simulink subsystem "dual_spin_omega_dot"  (R2023b)
settings: Solver=VariableStepAuto  StartTime=0.0  StopTime=10.0  RelTol=1e-3
libraries: matrix_library x1
settings Model: Creator=pierb  LastModifiedBy=pierb

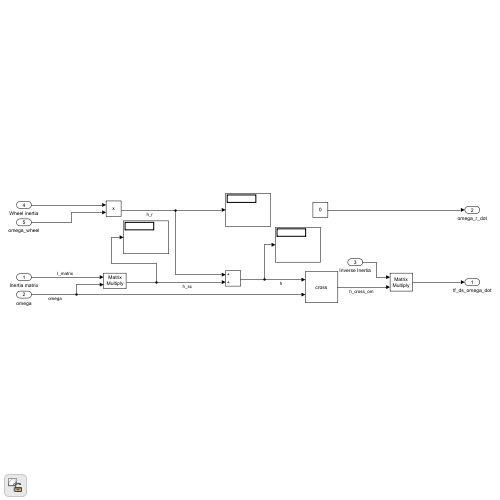
[thumbnail: Simulink's stored preview of the top-level diagram]
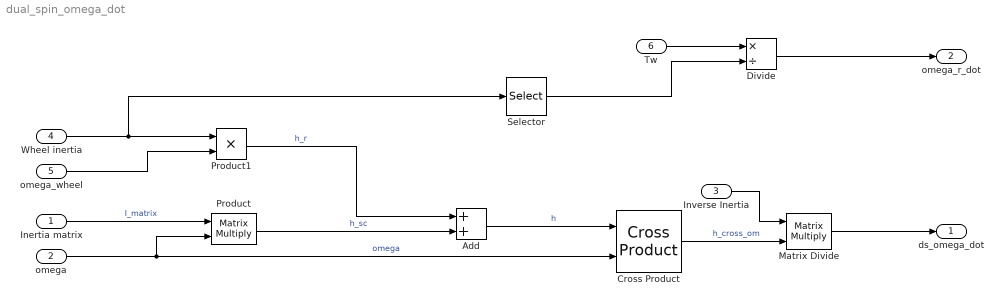
== system dual_spin_omega_dot ==
  Inertia matrix : Inport
  omega : Inport  Port=2
  Inverse Inertia : Inport  Port=3
  Wheel inertia : Inport  Port=4
  omega_wheel : Inport  Port=5
  Tw : Inport  Port=6
  Add : Sum
  Cross Product : matrix_library/Cross Product
  Divide : Product  Inputs=*/
  Matrix Divide : Product  Inputs=**  Multiplication=Matrix(*)
  Product : Product  Multiplication=Matrix(*)
  Product1 : Product
  Selector : Selector  InputPortWidth=3  IndexOptions=Index vector (dialog)  Indices=2  OutputSizes=1
  ds_omega_dot : Outport
  omega_r_dot : Outport  Port=2
  wires:
  Product1/1 -> Add/1  "h_r"
  omega/1 -> Product/2, Cross Product/2  "omega"
  Cross Product/1 -> Matrix Divide/2  "h_cross_om"
  Inverse Inertia/1 -> Matrix Divide/1
  omega_wheel/1 -> Product1/2
  Wheel inertia/1 -> Product1/1, Selector/1
  Add/1 -> Cross Product/1  "h"
  Inertia matrix/1 -> Product/1  "I_matrix"
  Product/1 -> Add/2  "h_sc"
  Matrix Divide/1 -> ds_omega_dot/1
  Tw/1 -> Divide/1
  Divide/1 -> omega_r_dot/1
  Selector/1 -> Divide/2
